simulink model "Project1_Final_Option2"  (R2023b)
settings: Solver=VariableStepAuto  StartTime=0.0  StopTime=10.0  RelTol=1e-3
values from neighbouring files (symbols this model uses):
  A = A_a(2)    [Project1.m]    (also in Project1_and_graphing.m; Project1_and_graphing_plz_check.m; Project1_week1.m = 4; Project1_week2.m = [0, 100])
  b = b_a(q)    [Project1.m]    (also in Project1_and_graphing.m; Project1_and_graphing_plz_check.m; Project1_week1.m = 1; Project1_week2.m = [10, 0.1])
  freq = freq_a(p)    [Project1.m]    (also in Project1_and_graphing.m; Project1_and_graphing_plz_check.m)
  J = J_a(r)    [Project1.m]    (also in Project1_and_graphing.m; Project1_and_graphing_plz_check.m; Project1_week1.m = 1; Project1_week2.m = [100, 0.01])
  sin_check = sin_check_a(k)    [Project1.m]    (also in Project1_and_graphing.m; Project1_and_graphing_plz_check.m)
settings Model: Creator=vince  LastModifiedBy=vince

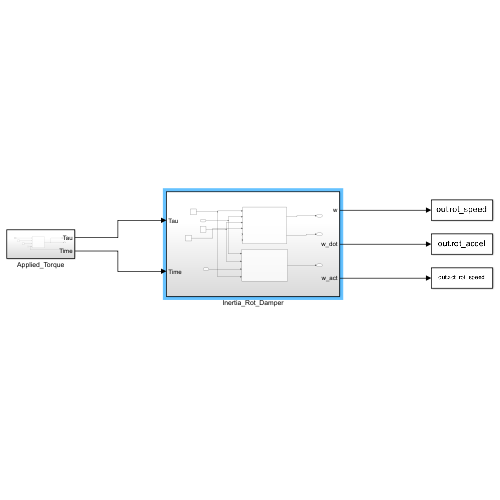
[thumbnail: Simulink's stored preview of the top-level diagram]
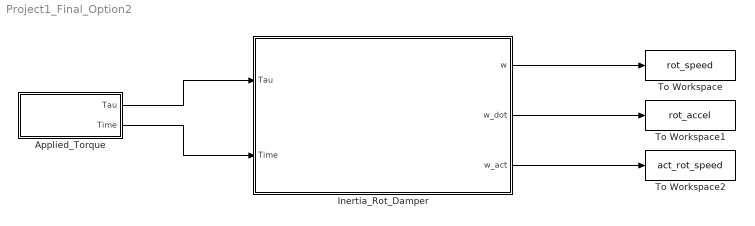
== system Project1_Final_Option2 ==
  Applied_Torque : Subsystem
  Inertia_Rot_Damper : Subsystem
  To Workspace : ToWorkspace  VariableName=rot_speed  SaveFormat=Timeseries  SampleTime=-1
  To Workspace1 : ToWorkspace  VariableName=rot_accel  SaveFormat=Timeseries  SampleTime=-1
  To Workspace2 : ToWorkspace  VariableName=act_rot_speed  SaveFormat=Timeseries  SampleTime=-1
  wires:
  Inertia_Rot_Damper/2(w_dot) -> To Workspace1/1
  Applied_Torque/2(Time) -> Inertia_Rot_Damper/2(Time)
  Inertia_Rot_Damper/3(w_act) -> To Workspace2/1
  Applied_Torque/1(Tau) -> Inertia_Rot_Damper/1(Tau)
  Inertia_Rot_Damper/1(w) -> To Workspace/1

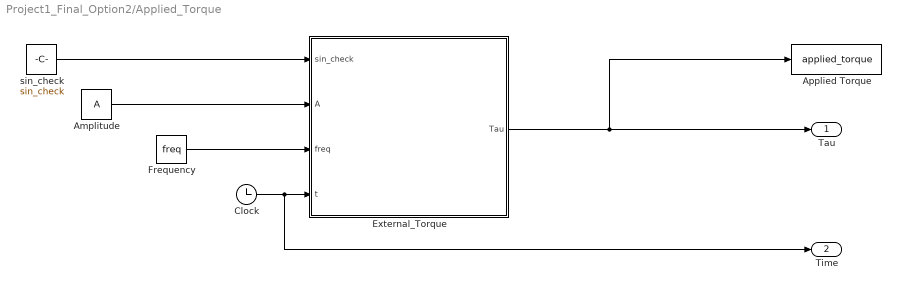
== system Project1_Final_Option2/Applied_Torque ==
  Amplitude : Constant  Value=A
  Applied Torque : ToWorkspace  VariableName=applied_torque  SaveFormat=Timeseries  SampleTime=-1
  Clock : Clock
      settings: Decimation=25
  External_Torque : MATLAB Function  TreatAsAtomicUnit=on
  Frequency : Constant  Value=freq
  sin_check : Constant  Value=sin_check
  Tau : Outport
  Time : Outport  Port=2
  wires:
  Frequency/1 -> External_Torque/3(freq)
  sin_check/1 -> External_Torque/1(sin_check)
  Amplitude/1 -> External_Torque/2(A)
  Clock/1 -> Time/1, External_Torque/4(t)
  External_Torque/1(Tau) -> Tau/1, Applied Torque/1

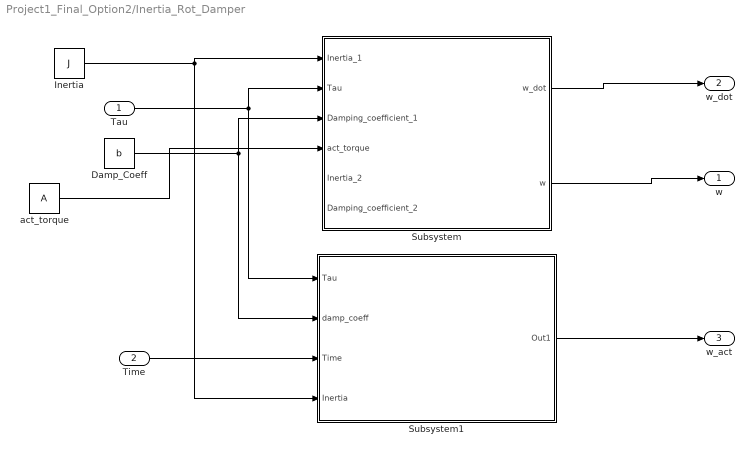
== system Project1_Final_Option2/Inertia_Rot_Damper ==
  Tau : Inport
  Time : Inport  Port=2
  Damp_Coeff : Constant  Value=b
  Inertia : Constant  Value=J
  Subsystem : Subsystem
  Subsystem1 : Subsystem
  act_torque : Constant  Value=A
  w : Outport
  w_dot : Outport  Port=2
  w_act : Outport  Port=3
  wires:
  Subsystem/2(w) -> w/1
  Subsystem/1(w_dot) -> w_dot/1
  Tau/1 -> Subsystem1/1(Tau), Subsystem/2(Tau)
  Inertia/1 -> Subsystem1/4(Inertia), Subsystem/1(Inertia_1)
  Damp_Coeff/1 -> Subsystem1/2(damp_coeff), Subsystem/3(Damping_coefficient_1)
  Subsystem1/1(Out1) -> w_act/1
  Time/1 -> Subsystem1/3(Time)
  act_torque/1 -> Subsystem/4(act_torque)

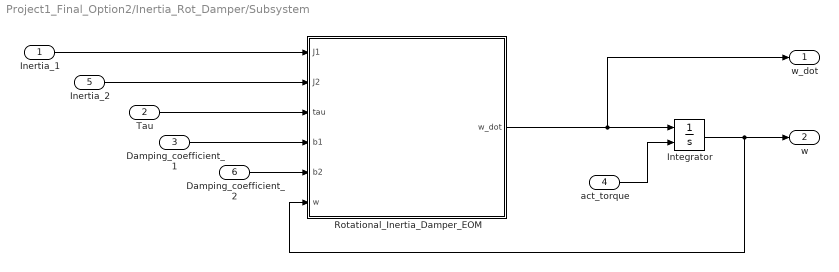
== system Project1_Final_Option2/Inertia_Rot_Damper/Subsystem ==
  Inertia_1 : Inport
  Tau : Inport  Port=2
  Damping_coefficient_1 : Inport  Port=3
  act_torque : Inport  Port=4
  Inertia_2 : Inport  Port=5
  Damping_coefficient_2 : Inport  Port=6
  Integrator : Integrator  InitialConditionSource=external
  Rotational_Inertia_Damper_EOM : MATLAB Function  TreatAsAtomicUnit=on
  w_dot : Outport
  w : Outport  Port=2
  wires:
  Integrator/1 -> Rotational_Inertia_Damper_EOM/6(w), w/1
  Inertia_1/1 -> Rotational_Inertia_Damper_EOM/1(J1)
  Rotational_Inertia_Damper_EOM/1(w_dot) -> w_dot/1, Integrator/1
  Tau/1 -> Rotational_Inertia_Damper_EOM/3(tau)
  act_torque/1 -> Integrator/2
  Inertia_2/1 -> Rotational_Inertia_Damper_EOM/2(J2)
  Damping_coefficient_1/1 -> Rotational_Inertia_Damper_EOM/4(b1)
  Damping_coefficient_2/1 -> Rotational_Inertia_Damper_EOM/5(b2)

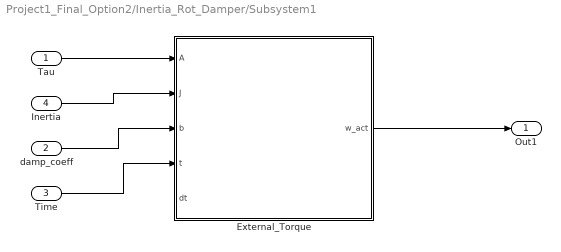
== system Project1_Final_Option2/Inertia_Rot_Damper/Subsystem1 ==
  Tau : Inport
  damp_coeff : Inport  Port=2
  Time : Inport  Port=3
  Inertia : Inport  Port=4
  External_Torque : MATLAB Function  TreatAsAtomicUnit=on
  Out1 : Outport
  wires:
  External_Torque/1(w_act) -> Out1/1
  Tau/1 -> External_Torque/1(A)
  Inertia/1 -> External_Torque/2(J)
  damp_coeff/1 -> External_Torque/3(b)
  Time/1 -> External_Torque/4(t)

== matlab function Project1_Final_Option2/Inertia_Rot_Damper/Subsystem/Rotational_Inertia_Damper_EOM ==
  data: J1 input; J2 input; tau input; b1 input; b2 input; w_dot output; w input
function w_dot = fcn(J1, J2, tau, b1, b2, w)
% Recall EOM: J*w_dot = tau_applied - tau_damped
tau_damped = (b1+b2)*w;
w_dot = (1/(J1+J2))*(tau - tau_damped);
end

== matlab function Project1_Final_Option2/Applied_Torque/External_Torque ==
  data: sin_check input; Tau output; A input; freq input; t input
function Tau = fcn(sin_check, A, freq, t)

if (sin_check == 0)
    Tau = A;

else 
    Tau = A*sin(freq*t);
end

== matlab function Project1_Final_Option2/Inertia_Rot_Damper/Subsystem1/External_Torque ==
  data: w_act output; A input; J input; b input; t input; dt input
function w_act = fcn(A, J, b, t, dt)

w_act = zeros(size(t));

% Initial condition
w_act(1) = 0; 

% Compute angular velocity over time
for i = 2:length(t)
    % Compute angular acceleration
    alpha = (A - b * w_act(i-1)) / J;
    
    % Update angular velocity
    w_act(i) = w_act(i-1) + alpha * dt;
end
